simulink library "ammclib_bam_S32K14x"  (R2016a)
settings: Solver=VariableStepAuto  SolverMode=SingleTasking  StartTime=0.0  StopTime=10.0  RelTol=1e-3
undefined symbols (not defined in the file or in its folder): f16A1, f16A2, f16ADCMaxError, f16B0, f16B1, f16B2, f16C1, f16CC1, f16CC1sc, f16CC1sc_D, f16CC1sc_Q, f16CC2, f16CC2sc, f16CC2sc_D, f16CC2sc_Q, f16DerivGain, f16EGain, f16FiltCoef, f16HystOff, f16HystOn, f16IGain, f16IntegGain, f16IntegGainFW, f16IntegGainQ, f16Kd, f16Kq, f16Limit, f16LowerLimit, f16LowerLimit_D, f16LowerLimit_Q, f16LowerLimitFW, f16LowerLimitQ, f16ModIndex, f16OutValOff, f16OutValOn, f16PropGain, f16PropGainFW, f16PropGainQ, f16RampDown, f16RampUp, f16UGain, f16UpperLimit, f16UpperLimit_D, f16UpperLimit_Q, f16UpperLimitFW, f16UpperLimitQ, f16WIGain, f32A1, f32A2, f32ADCMaxError, f32B0, f32B1, f32B2, f32C1, f32CC1, f32CC1sc, f32CC1sc_D, f32CC1sc_Q, f32CC2, f32CC2sc ... (+114)
(part 22 of 22)

== system ammclib_bam_S32K14x/MLIB/FLT/MLIB_Sub_FLT ==
  fltIn1 : Inport  OutDataTypeStr=single
  fltIn2 : Inport  Port=2  OutDataTypeStr=single
  MLIB_Sub_SF : S-Function  FunctionName=MLIB_Sub_SF_FLT  SFunctionDeploymentMode=off  EnableBusSupport=off
  copyright : Subsystem
      mask Display: text(10,90,'FILE:');text(10,75,'DESRIPTION:');text(10,60,'COPYRIGHT:');text(10,45,'VERSION:');text(10,30,'DATE:')
  copyright2 : Subsystem
      mask Display: text(10,90,'MLIB_Sub_BAM_FLT.mdl');text(10,75,'Subtraction.');text(10,60,'NXP 2020');text(10,45,'1.0');text(10,30,'18-Mar-2020');
  fltOut : Outport
  wires:
  MLIB_Sub_SF/1 -> fltOut/1
  fltIn2/1 -> MLIB_Sub_SF/2
  fltIn1/1 -> MLIB_Sub_SF/1

== system ammclib_bam_S32K14x/MLIB/FLT/MLIB_VAdd_FLT ==
  fltIn1 : Inport  OutDataTypeStr=Bus: SWLIBS_2Syst_FLT  BusOutputAsStruct=on
  fltIn2 : Inport  Port=2  OutDataTypeStr=Bus: SWLIBS_2Syst_FLT  BusOutputAsStruct=on
  MLIB_VAdd_SF : S-Function  FunctionName=MLIB_VAdd_SF_FLT  SFunctionDeploymentMode=off  EnableBusSupport=off
  copyright : Subsystem
      mask Display: text(10,90,'FILE:');text(10,75,'DESRIPTION:');text(10,60,'COPYRIGHT:');text(10,45,'VERSION:');text(10,30,'DATE:')
  copyright2 : Subsystem
      mask Display: text(10,90,'MLIB_VAdd_BAM_FLT.mdl');text(10,75,'Vector addition.');text(10,60,'NXP 2020');text(10,45,'1.0');text(10,30,'28-May-2020');
  fltOut : Outport
  wires:
  MLIB_VAdd_SF/1 -> fltOut/1
  fltIn2/1 -> MLIB_VAdd_SF/2
  fltIn1/1 -> MLIB_VAdd_SF/1

== system ammclib_bam_S32K14x/MLIB/FLT/MLIB_VMac_FLT ==
  fltIn1 : Inport  OutDataTypeStr=single
  fltIn2 : Inport  Port=2  OutDataTypeStr=single
  fltIn3 : Inport  Port=3  OutDataTypeStr=single
  fltIn4 : Inport  Port=4  OutDataTypeStr=single
  MLIB_VMac_SF : S-Function  FunctionName=MLIB_VMac_SF_FLT  SFunctionDeploymentMode=off  EnableBusSupport=off
  copyright : Subsystem
      mask Display: text(10,90,'FILE:');text(10,75,'DESRIPTION:');text(10,60,'COPYRIGHT:');text(10,45,'VERSION:');text(10,30,'DATE:')
  copyright2 : Subsystem
      mask Display: text(10,90,'MLIB_VMac_BAM_FLT.mdl');text(10,75,'Dot product of 2-element vectors.');text(10,60,'NXP 2020');text(10,45,'1.0');text(10,30,'18-Mar-2020');
  fltOut : Outport
  wires:
  MLIB_VMac_SF/1 -> fltOut/1
  fltIn4/1 -> MLIB_VMac_SF/4
  fltIn3/1 -> MLIB_VMac_SF/3
  fltIn2/1 -> MLIB_VMac_SF/2
  fltIn1/1 -> MLIB_VMac_SF/1

== system ammclib_bam_S32K14x/MLIB/FLT/MLIB_VScale_FLT ==
  fltInVec : Inport  OutDataTypeStr=Bus: SWLIBS_2Syst_FLT  BusOutputAsStruct=on
  fltInScale : Inport  Port=2  OutDataTypeStr=single
  MLIB_VScale_SF : S-Function  FunctionName=MLIB_VScale_SF_FLT  SFunctionDeploymentMode=off  EnableBusSupport=off
  copyright : Subsystem
      mask Display: text(10,90,'FILE:');text(10,75,'DESRIPTION:');text(10,60,'COPYRIGHT:');text(10,45,'VERSION:');text(10,30,'DATE:')
  copyright2 : Subsystem
      mask Display: text(10,90,'MLIB_VScale_BAM_FLT.mdl');text(10,75,'Multiplication of a vector and scalar.');text(10,60,'NXP 2020');text(10,45,'1.0');text(10,30,'03-Jun-2020');
  fltOutVec : Outport
  wires:
  MLIB_VScale_SF/1 -> fltOutVec/1
  fltInScale/1 -> MLIB_VScale_SF/2
  fltInVec/1 -> MLIB_VScale_SF/1

== system ammclib_bam_S32K14x/MLIB/FLT/MLIB_VSub_FLT ==
  fltIn1 : Inport  OutDataTypeStr=Bus: SWLIBS_2Syst_FLT  BusOutputAsStruct=on
  fltIn2 : Inport  Port=2  OutDataTypeStr=Bus: SWLIBS_2Syst_FLT  BusOutputAsStruct=on
  MLIB_VSub_SF : S-Function  FunctionName=MLIB_VSub_SF_FLT  SFunctionDeploymentMode=off  EnableBusSupport=off
  copyright : Subsystem
      mask Display: text(10,90,'FILE:');text(10,75,'DESRIPTION:');text(10,60,'COPYRIGHT:');text(10,45,'VERSION:');text(10,30,'DATE:')
  copyright2 : Subsystem
      mask Display: text(10,90,'MLIB_VSub_BAM_FLT.mdl');text(10,75,'Vector substraction.');text(10,60,'NXP 2020');text(10,45,'1.0');text(10,30,'01-Jun-2020');
  fltOut : Outport
  wires:
  MLIB_VSub_SF/1 -> fltOut/1
  fltIn2/1 -> MLIB_VSub_SF/2
  fltIn1/1 -> MLIB_VSub_SF/1

== system ammclib_bam_S32K14x/AMCLIB/F16/AMCLIB_BemfObsrvDQ_F16/copyright ==

== system ammclib_bam_S32K14x/AMCLIB/F16/AMCLIB_BemfObsrvDQ_F16/copyright2 ==

== system ammclib_bam_S32K14x/AMCLIB/F16/AMCLIB_CurrentLoop_F16/copyright ==

== system ammclib_bam_S32K14x/AMCLIB/F16/AMCLIB_CurrentLoop_F16/copyright2 ==

== system ammclib_bam_S32K14x/AMCLIB/F16/AMCLIB_FWSpeedLoop_F16/copyright ==

== system ammclib_bam_S32K14x/AMCLIB/F16/AMCLIB_FWSpeedLoop_F16/copyright2 ==

== system ammclib_bam_S32K14x/AMCLIB/F16/AMCLIB_FW_F16/copyright ==

== system ammclib_bam_S32K14x/AMCLIB/F16/AMCLIB_FW_F16/copyright2 ==

== system ammclib_bam_S32K14x/AMCLIB/F16/AMCLIB_SpeedLoop_F16/copyright ==

== system ammclib_bam_S32K14x/AMCLIB/F16/AMCLIB_SpeedLoop_F16/copyright2 ==

== system ammclib_bam_S32K14x/AMCLIB/F16/AMCLIB_TrackObsrv_F16/copyright ==

== system ammclib_bam_S32K14x/AMCLIB/F16/AMCLIB_TrackObsrv_F16/copyright2 ==

== system ammclib_bam_S32K14x/AMCLIB/F16/AMCLIB_Windmilling_F16/copyright ==

== system ammclib_bam_S32K14x/AMCLIB/F16/AMCLIB_Windmilling_F16/copyright2 ==

== system ammclib_bam_S32K14x/AMCLIB/F32/AMCLIB_BemfObsrvDQ_F32/copyright ==

== system ammclib_bam_S32K14x/AMCLIB/F32/AMCLIB_BemfObsrvDQ_F32/copyright2 ==

== system ammclib_bam_S32K14x/AMCLIB/F32/AMCLIB_CurrentLoop_F32/copyright ==

== system ammclib_bam_S32K14x/AMCLIB/F32/AMCLIB_CurrentLoop_F32/copyright2 ==

== system ammclib_bam_S32K14x/AMCLIB/F32/AMCLIB_FWSpeedLoop_F32/copyright ==

== system ammclib_bam_S32K14x/AMCLIB/F32/AMCLIB_FWSpeedLoop_F32/copyright2 ==

== system ammclib_bam_S32K14x/AMCLIB/F32/AMCLIB_FW_F32/copyright ==

== system ammclib_bam_S32K14x/AMCLIB/F32/AMCLIB_FW_F32/copyright2 ==

== system ammclib_bam_S32K14x/AMCLIB/F32/AMCLIB_SpeedLoop_F32/copyright ==

== system ammclib_bam_S32K14x/AMCLIB/F32/AMCLIB_SpeedLoop_F32/copyright2 ==

== system ammclib_bam_S32K14x/AMCLIB/F32/AMCLIB_TrackObsrv_F32/copyright ==

== system ammclib_bam_S32K14x/AMCLIB/F32/AMCLIB_TrackObsrv_F32/copyright2 ==

== system ammclib_bam_S32K14x/AMCLIB/F32/AMCLIB_Windmilling_F32/copyright ==

== system ammclib_bam_S32K14x/AMCLIB/F32/AMCLIB_Windmilling_F32/copyright2 ==

== system ammclib_bam_S32K14x/AMCLIB/FLT/AMCLIB_BemfObsrvDQ_FLT/copyright ==

== system ammclib_bam_S32K14x/AMCLIB/FLT/AMCLIB_BemfObsrvDQ_FLT/copyright2 ==

== system ammclib_bam_S32K14x/AMCLIB/FLT/AMCLIB_CurrentLoop_FLT/copyright ==

== system ammclib_bam_S32K14x/AMCLIB/FLT/AMCLIB_CurrentLoop_FLT/copyright2 ==

== system ammclib_bam_S32K14x/AMCLIB/FLT/AMCLIB_FWSpeedLoop_FLT/copyright ==

== system ammclib_bam_S32K14x/AMCLIB/FLT/AMCLIB_FWSpeedLoop_FLT/copyright2 ==

== system ammclib_bam_S32K14x/AMCLIB/FLT/AMCLIB_FW_FLT/copyright ==

== system ammclib_bam_S32K14x/AMCLIB/FLT/AMCLIB_FW_FLT/copyright2 ==

== system ammclib_bam_S32K14x/AMCLIB/FLT/AMCLIB_SpeedLoop_FLT/copyright ==

== system ammclib_bam_S32K14x/AMCLIB/FLT/AMCLIB_SpeedLoop_FLT/copyright2 ==

== system ammclib_bam_S32K14x/AMCLIB/FLT/AMCLIB_TrackObsrv_FLT/copyright ==

== system ammclib_bam_S32K14x/AMCLIB/FLT/AMCLIB_TrackObsrv_FLT/copyright2 ==

== system ammclib_bam_S32K14x/AMCLIB/FLT/AMCLIB_Windmilling_FLT/copyright ==

== system ammclib_bam_S32K14x/AMCLIB/FLT/AMCLIB_Windmilling_FLT/copyright2 ==

== system ammclib_bam_S32K14x/GDFLIB/F16/GDFLIB_FilterFIR_F16/copyright ==

== system ammclib_bam_S32K14x/GDFLIB/F16/GDFLIB_FilterFIR_F16/copyright2 ==

== system ammclib_bam_S32K14x/GDFLIB/F16/GDFLIB_FilterIIR1_F16/copyright ==

== system ammclib_bam_S32K14x/GDFLIB/F16/GDFLIB_FilterIIR1_F16/copyright2 ==

== system ammclib_bam_S32K14x/GDFLIB/F16/GDFLIB_FilterIIR2_F16/copyright ==

== system ammclib_bam_S32K14x/GDFLIB/F16/GDFLIB_FilterIIR2_F16/copyright2 ==

== system ammclib_bam_S32K14x/GDFLIB/F16/GDFLIB_FilterMA_F16/copyright ==

== system ammclib_bam_S32K14x/GDFLIB/F16/GDFLIB_FilterMA_F16/copyright2 ==

== system ammclib_bam_S32K14x/GDFLIB/F32/GDFLIB_FilterFIR_F32/copyright ==

== system ammclib_bam_S32K14x/GDFLIB/F32/GDFLIB_FilterFIR_F32/copyright2 ==

== system ammclib_bam_S32K14x/GDFLIB/F32/GDFLIB_FilterIIR1_F32/copyright ==

== system ammclib_bam_S32K14x/GDFLIB/F32/GDFLIB_FilterIIR1_F32/copyright2 ==

== system ammclib_bam_S32K14x/GDFLIB/F32/GDFLIB_FilterIIR2_F32/copyright ==

== system ammclib_bam_S32K14x/GDFLIB/F32/GDFLIB_FilterIIR2_F32/copyright2 ==

== system ammclib_bam_S32K14x/GDFLIB/F32/GDFLIB_FilterMA_F32/copyright ==

== system ammclib_bam_S32K14x/GDFLIB/F32/GDFLIB_FilterMA_F32/copyright2 ==

== system ammclib_bam_S32K14x/GDFLIB/FLT/GDFLIB_FilterFIR_FLT/copyright ==

== system ammclib_bam_S32K14x/GDFLIB/FLT/GDFLIB_FilterFIR_FLT/copyright2 ==

== system ammclib_bam_S32K14x/GDFLIB/FLT/GDFLIB_FilterIIR1_FLT/copyright ==

== system ammclib_bam_S32K14x/GDFLIB/FLT/GDFLIB_FilterIIR1_FLT/copyright2 ==

== system ammclib_bam_S32K14x/GDFLIB/FLT/GDFLIB_FilterIIR2_FLT/copyright ==

== system ammclib_bam_S32K14x/GDFLIB/FLT/GDFLIB_FilterIIR2_FLT/copyright2 ==

== system ammclib_bam_S32K14x/GDFLIB/FLT/GDFLIB_FilterMA_FLT/copyright ==

== system ammclib_bam_S32K14x/GDFLIB/FLT/GDFLIB_FilterMA_FLT/copyright2 ==

== system ammclib_bam_S32K14x/GFLIB/F16/GFLIB_Acos_F16/copyright ==

== system ammclib_bam_S32K14x/GFLIB/F16/GFLIB_Acos_F16/copyright2 ==

== system ammclib_bam_S32K14x/GFLIB/F16/GFLIB_Asin_F16/copyright ==

== system ammclib_bam_S32K14x/GFLIB/F16/GFLIB_Asin_F16/copyright2 ==

== system ammclib_bam_S32K14x/GFLIB/F16/GFLIB_AtanYXShifted_F16/copyright ==

== system ammclib_bam_S32K14x/GFLIB/F16/GFLIB_AtanYXShifted_F16/copyright2 ==

== system ammclib_bam_S32K14x/GFLIB/F16/GFLIB_AtanYX_F16/copyright ==

== system ammclib_bam_S32K14x/GFLIB/F16/GFLIB_AtanYX_F16/copyright2 ==

== system ammclib_bam_S32K14x/GFLIB/F16/GFLIB_Atan_F16/copyright ==

== system ammclib_bam_S32K14x/GFLIB/F16/GFLIB_Atan_F16/copyright2 ==

== system ammclib_bam_S32K14x/GFLIB/F16/GFLIB_ControllerPIDpAW_F16/copyright ==

== system ammclib_bam_S32K14x/GFLIB/F16/GFLIB_ControllerPIDpAW_F16/copyright2 ==

== system ammclib_bam_S32K14x/GFLIB/F16/GFLIB_ControllerPIpAW_F16/copyright ==

== system ammclib_bam_S32K14x/GFLIB/F16/GFLIB_ControllerPIpAW_F16/copyright2 ==

== system ammclib_bam_S32K14x/GFLIB/F16/GFLIB_ControllerPIp_F16/copyright ==

== system ammclib_bam_S32K14x/GFLIB/F16/GFLIB_ControllerPIp_F16/copyright2 ==

== system ammclib_bam_S32K14x/GFLIB/F16/GFLIB_ControllerPIrAW_F16/copyright ==

== system ammclib_bam_S32K14x/GFLIB/F16/GFLIB_ControllerPIrAW_F16/copyright2 ==

== system ammclib_bam_S32K14x/GFLIB/F16/GFLIB_ControllerPIr_F16/copyright ==

== system ammclib_bam_S32K14x/GFLIB/F16/GFLIB_ControllerPIr_F16/copyright2 ==

== system ammclib_bam_S32K14x/GFLIB/F16/GFLIB_Cos_F16/copyright ==

== system ammclib_bam_S32K14x/GFLIB/F16/GFLIB_Cos_F16/copyright2 ==

== system ammclib_bam_S32K14x/GFLIB/F16/GFLIB_Hyst_F16/copyright ==

== system ammclib_bam_S32K14x/GFLIB/F16/GFLIB_Hyst_F16/copyright2 ==

== system ammclib_bam_S32K14x/GFLIB/F16/GFLIB_IntegratorTR_F16/copyright ==

== system ammclib_bam_S32K14x/GFLIB/F16/GFLIB_IntegratorTR_F16/copyright2 ==

== system ammclib_bam_S32K14x/GFLIB/F16/GFLIB_Limit_F16/copyright ==

== system ammclib_bam_S32K14x/GFLIB/F16/GFLIB_Limit_F16/copyright2 ==

== system ammclib_bam_S32K14x/GFLIB/F16/GFLIB_LowerLimit_F16/copyright ==

== system ammclib_bam_S32K14x/GFLIB/F16/GFLIB_LowerLimit_F16/copyright2 ==

== system ammclib_bam_S32K14x/GFLIB/F16/GFLIB_Lut1D_F16/copyright ==

== system ammclib_bam_S32K14x/GFLIB/F16/GFLIB_Lut1D_F16/copyright2 ==

== system ammclib_bam_S32K14x/GFLIB/F16/GFLIB_Lut2D_F16/copyright ==

== system ammclib_bam_S32K14x/GFLIB/F16/GFLIB_Lut2D_F16/copyright2 ==

== system ammclib_bam_S32K14x/GFLIB/F16/GFLIB_Ramp_F16/copyright ==

== system ammclib_bam_S32K14x/GFLIB/F16/GFLIB_Ramp_F16/copyright2 ==

== system ammclib_bam_S32K14x/GFLIB/F16/GFLIB_Sign_F16/copyright ==

== system ammclib_bam_S32K14x/GFLIB/F16/GFLIB_Sign_F16/copyright2 ==

== system ammclib_bam_S32K14x/GFLIB/F16/GFLIB_SinCos_F16/copyright ==

== system ammclib_bam_S32K14x/GFLIB/F16/GFLIB_SinCos_F16/copyright2 ==

== system ammclib_bam_S32K14x/GFLIB/F16/GFLIB_Sin_F16/copyright ==

== system ammclib_bam_S32K14x/GFLIB/F16/GFLIB_Sin_F16/copyright2 ==

== system ammclib_bam_S32K14x/GFLIB/F16/GFLIB_Sqrt_F16/copyright ==

== system ammclib_bam_S32K14x/GFLIB/F16/GFLIB_Sqrt_F16/copyright2 ==

== system ammclib_bam_S32K14x/GFLIB/F16/GFLIB_Tan_F16/copyright ==

== system ammclib_bam_S32K14x/GFLIB/F16/GFLIB_Tan_F16/copyright2 ==

== system ammclib_bam_S32K14x/GFLIB/F16/GFLIB_UpperLimit_F16/copyright ==

== system ammclib_bam_S32K14x/GFLIB/F16/GFLIB_UpperLimit_F16/copyright2 ==

== system ammclib_bam_S32K14x/GFLIB/F16/GFLIB_VMin_F16/copyright ==

== system ammclib_bam_S32K14x/GFLIB/F16/GFLIB_VMin_F16/copyright2 ==

== system ammclib_bam_S32K14x/GFLIB/F16/GFLIB_VectorLimit_F16/copyright ==

== system ammclib_bam_S32K14x/GFLIB/F16/GFLIB_VectorLimit_F16/copyright2 ==

== system ammclib_bam_S32K14x/GFLIB/F32/GFLIB_Acos_F32/copyright ==

== system ammclib_bam_S32K14x/GFLIB/F32/GFLIB_Acos_F32/copyright2 ==

== system ammclib_bam_S32K14x/GFLIB/F32/GFLIB_Asin_F32/copyright ==

== system ammclib_bam_S32K14x/GFLIB/F32/GFLIB_Asin_F32/copyright2 ==

== system ammclib_bam_S32K14x/GFLIB/F32/GFLIB_AtanYXShifted_F32/copyright ==

== system ammclib_bam_S32K14x/GFLIB/F32/GFLIB_AtanYXShifted_F32/copyright2 ==

== system ammclib_bam_S32K14x/GFLIB/F32/GFLIB_AtanYX_F32/copyright ==

== system ammclib_bam_S32K14x/GFLIB/F32/GFLIB_AtanYX_F32/copyright2 ==

== system ammclib_bam_S32K14x/GFLIB/F32/GFLIB_Atan_F32/copyright ==

== system ammclib_bam_S32K14x/GFLIB/F32/GFLIB_Atan_F32/copyright2 ==

== system ammclib_bam_S32K14x/GFLIB/F32/GFLIB_ControllerPIDpAW_F32/copyright ==

== system ammclib_bam_S32K14x/GFLIB/F32/GFLIB_ControllerPIDpAW_F32/copyright2 ==

== system ammclib_bam_S32K14x/GFLIB/F32/GFLIB_ControllerPIpAW_F32/copyright ==

== system ammclib_bam_S32K14x/GFLIB/F32/GFLIB_ControllerPIpAW_F32/copyright2 ==

== system ammclib_bam_S32K14x/GFLIB/F32/GFLIB_ControllerPIp_F32/copyright ==

== system ammclib_bam_S32K14x/GFLIB/F32/GFLIB_ControllerPIp_F32/copyright2 ==

== system ammclib_bam_S32K14x/GFLIB/F32/GFLIB_ControllerPIrAW_F32/copyright ==

== system ammclib_bam_S32K14x/GFLIB/F32/GFLIB_ControllerPIrAW_F32/copyright2 ==

== system ammclib_bam_S32K14x/GFLIB/F32/GFLIB_ControllerPIr_F32/copyright ==

== system ammclib_bam_S32K14x/GFLIB/F32/GFLIB_ControllerPIr_F32/copyright2 ==

== system ammclib_bam_S32K14x/GFLIB/F32/GFLIB_Cos_F32/copyright ==

== system ammclib_bam_S32K14x/GFLIB/F32/GFLIB_Cos_F32/copyright2 ==

== system ammclib_bam_S32K14x/GFLIB/F32/GFLIB_Hyst_F32/copyright ==

== system ammclib_bam_S32K14x/GFLIB/F32/GFLIB_Hyst_F32/copyright2 ==

== system ammclib_bam_S32K14x/GFLIB/F32/GFLIB_IntegratorTR_F32/copyright ==

== system ammclib_bam_S32K14x/GFLIB/F32/GFLIB_IntegratorTR_F32/copyright2 ==

== system ammclib_bam_S32K14x/GFLIB/F32/GFLIB_Limit_F32/copyright ==

== system ammclib_bam_S32K14x/GFLIB/F32/GFLIB_Limit_F32/copyright2 ==

== system ammclib_bam_S32K14x/GFLIB/F32/GFLIB_LowerLimit_F32/copyright ==

== system ammclib_bam_S32K14x/GFLIB/F32/GFLIB_LowerLimit_F32/copyright2 ==

== system ammclib_bam_S32K14x/GFLIB/F32/GFLIB_Lut1D_F32/copyright ==

== system ammclib_bam_S32K14x/GFLIB/F32/GFLIB_Lut1D_F32/copyright2 ==

== system ammclib_bam_S32K14x/GFLIB/F32/GFLIB_Lut2D_F32/copyright ==

== system ammclib_bam_S32K14x/GFLIB/F32/GFLIB_Lut2D_F32/copyright2 ==

== system ammclib_bam_S32K14x/GFLIB/F32/GFLIB_Ramp_F32/copyright ==

== system ammclib_bam_S32K14x/GFLIB/F32/GFLIB_Ramp_F32/copyright2 ==

== system ammclib_bam_S32K14x/GFLIB/F32/GFLIB_Sign_F32/copyright ==

== system ammclib_bam_S32K14x/GFLIB/F32/GFLIB_Sign_F32/copyright2 ==

== system ammclib_bam_S32K14x/GFLIB/F32/GFLIB_SinCos_F32/copyright ==

== system ammclib_bam_S32K14x/GFLIB/F32/GFLIB_SinCos_F32/copyright2 ==

== system ammclib_bam_S32K14x/GFLIB/F32/GFLIB_Sin_F32/copyright ==

== system ammclib_bam_S32K14x/GFLIB/F32/GFLIB_Sin_F32/copyright2 ==

== system ammclib_bam_S32K14x/GFLIB/F32/GFLIB_Sqrt_F32/copyright ==

== system ammclib_bam_S32K14x/GFLIB/F32/GFLIB_Sqrt_F32/copyright2 ==

== system ammclib_bam_S32K14x/GFLIB/F32/GFLIB_Tan_F32/copyright ==

== system ammclib_bam_S32K14x/GFLIB/F32/GFLIB_Tan_F32/copyright2 ==

== system ammclib_bam_S32K14x/GFLIB/F32/GFLIB_UpperLimit_F32/copyright ==

== system ammclib_bam_S32K14x/GFLIB/F32/GFLIB_UpperLimit_F32/copyright2 ==

== system ammclib_bam_S32K14x/GFLIB/F32/GFLIB_VMin_F32/copyright ==

== system ammclib_bam_S32K14x/GFLIB/F32/GFLIB_VMin_F32/copyright2 ==

== system ammclib_bam_S32K14x/GFLIB/F32/GFLIB_VectorLimit_F32/copyright ==

== system ammclib_bam_S32K14x/GFLIB/F32/GFLIB_VectorLimit_F32/copyright2 ==

== system ammclib_bam_S32K14x/GFLIB/FLT/GFLIB_Acos_FLT/copyright ==

== system ammclib_bam_S32K14x/GFLIB/FLT/GFLIB_Acos_FLT/copyright2 ==

== system ammclib_bam_S32K14x/GFLIB/FLT/GFLIB_Asin_FLT/copyright ==

== system ammclib_bam_S32K14x/GFLIB/FLT/GFLIB_Asin_FLT/copyright2 ==

== system ammclib_bam_S32K14x/GFLIB/FLT/GFLIB_AtanYXShifted_FLT/copyright ==

== system ammclib_bam_S32K14x/GFLIB/FLT/GFLIB_AtanYXShifted_FLT/copyright2 ==

== system ammclib_bam_S32K14x/GFLIB/FLT/GFLIB_AtanYX_FLT/copyright ==

== system ammclib_bam_S32K14x/GFLIB/FLT/GFLIB_AtanYX_FLT/copyright2 ==

== system ammclib_bam_S32K14x/GFLIB/FLT/GFLIB_Atan_FLT/copyright ==

== system ammclib_bam_S32K14x/GFLIB/FLT/GFLIB_Atan_FLT/copyright2 ==

== system ammclib_bam_S32K14x/GFLIB/FLT/GFLIB_ControllerPIDpAW_FLT/copyright ==

== system ammclib_bam_S32K14x/GFLIB/FLT/GFLIB_ControllerPIDpAW_FLT/copyright2 ==

== system ammclib_bam_S32K14x/GFLIB/FLT/GFLIB_ControllerPIpAW_FLT/copyright ==

== system ammclib_bam_S32K14x/GFLIB/FLT/GFLIB_ControllerPIpAW_FLT/copyright2 ==

== system ammclib_bam_S32K14x/GFLIB/FLT/GFLIB_ControllerPIp_FLT/copyright ==

== system ammclib_bam_S32K14x/GFLIB/FLT/GFLIB_ControllerPIp_FLT/copyright2 ==

== system ammclib_bam_S32K14x/GFLIB/FLT/GFLIB_ControllerPIrAW_FLT/copyright ==

== system ammclib_bam_S32K14x/GFLIB/FLT/GFLIB_ControllerPIrAW_FLT/copyright2 ==

== system ammclib_bam_S32K14x/GFLIB/FLT/GFLIB_ControllerPIr_FLT/copyright ==

== system ammclib_bam_S32K14x/GFLIB/FLT/GFLIB_ControllerPIr_FLT/copyright2 ==

== system ammclib_bam_S32K14x/GFLIB/FLT/GFLIB_Cos_FLT/copyright ==

== system ammclib_bam_S32K14x/GFLIB/FLT/GFLIB_Cos_FLT/copyright2 ==

== system ammclib_bam_S32K14x/GFLIB/FLT/GFLIB_Hyst_FLT/copyright ==

== system ammclib_bam_S32K14x/GFLIB/FLT/GFLIB_Hyst_FLT/copyright2 ==

== system ammclib_bam_S32K14x/GFLIB/FLT/GFLIB_IntegratorTR_FLT/copyright ==

== system ammclib_bam_S32K14x/GFLIB/FLT/GFLIB_IntegratorTR_FLT/copyright2 ==

== system ammclib_bam_S32K14x/GFLIB/FLT/GFLIB_Limit_FLT/copyright ==

== system ammclib_bam_S32K14x/GFLIB/FLT/GFLIB_Limit_FLT/copyright2 ==

== system ammclib_bam_S32K14x/GFLIB/FLT/GFLIB_Log10_FLT/copyright ==

== system ammclib_bam_S32K14x/GFLIB/FLT/GFLIB_Log10_FLT/copyright2 ==

== system ammclib_bam_S32K14x/GFLIB/FLT/GFLIB_LowerLimit_FLT/copyright ==

== system ammclib_bam_S32K14x/GFLIB/FLT/GFLIB_LowerLimit_FLT/copyright2 ==

== system ammclib_bam_S32K14x/GFLIB/FLT/GFLIB_Lut1D_FLT/copyright ==

== system ammclib_bam_S32K14x/GFLIB/FLT/GFLIB_Lut1D_FLT/copyright2 ==

== system ammclib_bam_S32K14x/GFLIB/FLT/GFLIB_Lut2D_FLT/copyright ==

== system ammclib_bam_S32K14x/GFLIB/FLT/GFLIB_Lut2D_FLT/copyright2 ==

== system ammclib_bam_S32K14x/GFLIB/FLT/GFLIB_Ramp_FLT/copyright ==

== system ammclib_bam_S32K14x/GFLIB/FLT/GFLIB_Ramp_FLT/copyright2 ==

== system ammclib_bam_S32K14x/GFLIB/FLT/GFLIB_Sign_FLT/copyright ==

== system ammclib_bam_S32K14x/GFLIB/FLT/GFLIB_Sign_FLT/copyright2 ==

== system ammclib_bam_S32K14x/GFLIB/FLT/GFLIB_SinCos_FLT/copyright ==

== system ammclib_bam_S32K14x/GFLIB/FLT/GFLIB_SinCos_FLT/copyright2 ==

== system ammclib_bam_S32K14x/GFLIB/FLT/GFLIB_Sin_FLT/copyright ==

== system ammclib_bam_S32K14x/GFLIB/FLT/GFLIB_Sin_FLT/copyright2 ==

== system ammclib_bam_S32K14x/GFLIB/FLT/GFLIB_Sqrt_FLT/copyright ==

== system ammclib_bam_S32K14x/GFLIB/FLT/GFLIB_Sqrt_FLT/copyright2 ==

== system ammclib_bam_S32K14x/GFLIB/FLT/GFLIB_Tan_FLT/copyright ==

== system ammclib_bam_S32K14x/GFLIB/FLT/GFLIB_Tan_FLT/copyright2 ==

== system ammclib_bam_S32K14x/GFLIB/FLT/GFLIB_UpperLimit_FLT/copyright ==

== system ammclib_bam_S32K14x/GFLIB/FLT/GFLIB_UpperLimit_FLT/copyright2 ==

== system ammclib_bam_S32K14x/GFLIB/FLT/GFLIB_VLog10_FLT/copyright ==

== system ammclib_bam_S32K14x/GFLIB/FLT/GFLIB_VLog10_FLT/copyright2 ==

== system ammclib_bam_S32K14x/GFLIB/FLT/GFLIB_VMin_FLT/copyright ==

== system ammclib_bam_S32K14x/GFLIB/FLT/GFLIB_VMin_FLT/copyright2 ==

== system ammclib_bam_S32K14x/GFLIB/FLT/GFLIB_VectorLimit_FLT/copyright ==

== system ammclib_bam_S32K14x/GFLIB/FLT/GFLIB_VectorLimit_FLT/copyright2 ==

== system ammclib_bam_S32K14x/GMCLIB/F16/GMCLIB_BetaProjection3Ph_F16/copyright ==

== system ammclib_bam_S32K14x/GMCLIB/F16/GMCLIB_BetaProjection3Ph_F16/copyright2 ==

== system ammclib_bam_S32K14x/GMCLIB/F16/GMCLIB_BetaProjection_F16/copyright ==

== system ammclib_bam_S32K14x/GMCLIB/F16/GMCLIB_BetaProjection_F16/copyright2 ==

== system ammclib_bam_S32K14x/GMCLIB/F16/GMCLIB_ClarkInv_F16/copyright ==

== system ammclib_bam_S32K14x/GMCLIB/F16/GMCLIB_ClarkInv_F16/copyright2 ==

== system ammclib_bam_S32K14x/GMCLIB/F16/GMCLIB_Clark_F16/copyright ==

== system ammclib_bam_S32K14x/GMCLIB/F16/GMCLIB_Clark_F16/copyright2 ==

== system ammclib_bam_S32K14x/GMCLIB/F16/GMCLIB_DecouplingPMSM_F16/copyright ==

== system ammclib_bam_S32K14x/GMCLIB/F16/GMCLIB_DecouplingPMSM_F16/copyright2 ==

== system ammclib_bam_S32K14x/GMCLIB/F16/GMCLIB_ElimDcBusRip_F16/copyright ==

== system ammclib_bam_S32K14x/GMCLIB/F16/GMCLIB_ElimDcBusRip_F16/copyright2 ==

== system ammclib_bam_S32K14x/GMCLIB/F16/GMCLIB_ParkInv_F16/copyright ==

== system ammclib_bam_S32K14x/GMCLIB/F16/GMCLIB_ParkInv_F16/copyright2 ==

== system ammclib_bam_S32K14x/GMCLIB/F16/GMCLIB_Park_F16/copyright ==

== system ammclib_bam_S32K14x/GMCLIB/F16/GMCLIB_Park_F16/copyright2 ==

== system ammclib_bam_S32K14x/GMCLIB/F16/GMCLIB_PwmIct_F16/copyright ==

== system ammclib_bam_S32K14x/GMCLIB/F16/GMCLIB_PwmIct_F16/copyright2 ==

== system ammclib_bam_S32K14x/GMCLIB/F16/GMCLIB_SvmSci_F16/copyright ==

== system ammclib_bam_S32K14x/GMCLIB/F16/GMCLIB_SvmSci_F16/copyright2 ==

== system ammclib_bam_S32K14x/GMCLIB/F16/GMCLIB_SvmStd_F16/copyright ==

== system ammclib_bam_S32K14x/GMCLIB/F16/GMCLIB_SvmStd_F16/copyright2 ==

== system ammclib_bam_S32K14x/GMCLIB/F16/GMCLIB_SvmU0n_F16/copyright ==

== system ammclib_bam_S32K14x/GMCLIB/F16/GMCLIB_SvmU0n_F16/copyright2 ==

== system ammclib_bam_S32K14x/GMCLIB/F16/GMCLIB_SvmU7n_F16/copyright ==

== system ammclib_bam_S32K14x/GMCLIB/F16/GMCLIB_SvmU7n_F16/copyright2 ==

== system ammclib_bam_S32K14x/GMCLIB/F16/GMCLIB_VRot_F16/copyright ==

== system ammclib_bam_S32K14x/GMCLIB/F16/GMCLIB_VRot_F16/copyright2 ==

== system ammclib_bam_S32K14x/GMCLIB/F16/GMCLIB_VUnit_F16/copyright ==

== system ammclib_bam_S32K14x/GMCLIB/F16/GMCLIB_VUnit_F16/copyright2 ==

== system ammclib_bam_S32K14x/GMCLIB/F16/GMCLIB_Vpol2xy_F16/copyright ==

== system ammclib_bam_S32K14x/GMCLIB/F16/GMCLIB_Vpol2xy_F16/copyright2 ==

== system ammclib_bam_S32K14x/GMCLIB/F16/GMCLIB_Vxy2pol_F16/copyright ==

== system ammclib_bam_S32K14x/GMCLIB/F16/GMCLIB_Vxy2pol_F16/copyright2 ==

== system ammclib_bam_S32K14x/GMCLIB/F32/GMCLIB_BetaProjection3Ph_F32/copyright ==

== system ammclib_bam_S32K14x/GMCLIB/F32/GMCLIB_BetaProjection3Ph_F32/copyright2 ==

== system ammclib_bam_S32K14x/GMCLIB/F32/GMCLIB_BetaProjection_F32/copyright ==

== system ammclib_bam_S32K14x/GMCLIB/F32/GMCLIB_BetaProjection_F32/copyright2 ==

== system ammclib_bam_S32K14x/GMCLIB/F32/GMCLIB_ClarkInv_F32/copyright ==

== system ammclib_bam_S32K14x/GMCLIB/F32/GMCLIB_ClarkInv_F32/copyright2 ==

== system ammclib_bam_S32K14x/GMCLIB/F32/GMCLIB_Clark_F32/copyright ==

== system ammclib_bam_S32K14x/GMCLIB/F32/GMCLIB_Clark_F32/copyright2 ==

== system ammclib_bam_S32K14x/GMCLIB/F32/GMCLIB_DecouplingPMSM_F32/copyright ==

== system ammclib_bam_S32K14x/GMCLIB/F32/GMCLIB_DecouplingPMSM_F32/copyright2 ==

== system ammclib_bam_S32K14x/GMCLIB/F32/GMCLIB_ElimDcBusRip_F32/copyright ==

== system ammclib_bam_S32K14x/GMCLIB/F32/GMCLIB_ElimDcBusRip_F32/copyright2 ==

== system ammclib_bam_S32K14x/GMCLIB/F32/GMCLIB_ParkInv_F32/copyright ==

== system ammclib_bam_S32K14x/GMCLIB/F32/GMCLIB_ParkInv_F32/copyright2 ==

== system ammclib_bam_S32K14x/GMCLIB/F32/GMCLIB_Park_F32/copyright ==

== system ammclib_bam_S32K14x/GMCLIB/F32/GMCLIB_Park_F32/copyright2 ==

== system ammclib_bam_S32K14x/GMCLIB/F32/GMCLIB_PwmIct_F32/copyright ==

== system ammclib_bam_S32K14x/GMCLIB/F32/GMCLIB_PwmIct_F32/copyright2 ==

== system ammclib_bam_S32K14x/GMCLIB/F32/GMCLIB_SvmSci_F32/copyright ==

== system ammclib_bam_S32K14x/GMCLIB/F32/GMCLIB_SvmSci_F32/copyright2 ==

== system ammclib_bam_S32K14x/GMCLIB/F32/GMCLIB_SvmStd_F32/copyright ==

== system ammclib_bam_S32K14x/GMCLIB/F32/GMCLIB_SvmStd_F32/copyright2 ==

== system ammclib_bam_S32K14x/GMCLIB/F32/GMCLIB_SvmU0n_F32/copyright ==

== system ammclib_bam_S32K14x/GMCLIB/F32/GMCLIB_SvmU0n_F32/copyright2 ==

== system ammclib_bam_S32K14x/GMCLIB/F32/GMCLIB_SvmU7n_F32/copyright ==

== system ammclib_bam_S32K14x/GMCLIB/F32/GMCLIB_SvmU7n_F32/copyright2 ==

== system ammclib_bam_S32K14x/GMCLIB/F32/GMCLIB_VRot_F32/copyright ==

== system ammclib_bam_S32K14x/GMCLIB/F32/GMCLIB_VRot_F32/copyright2 ==

== system ammclib_bam_S32K14x/GMCLIB/F32/GMCLIB_VUnit_F32/copyright ==

== system ammclib_bam_S32K14x/GMCLIB/F32/GMCLIB_VUnit_F32/copyright2 ==

== system ammclib_bam_S32K14x/GMCLIB/F32/GMCLIB_Vpol2xy_F32/copyright ==

== system ammclib_bam_S32K14x/GMCLIB/F32/GMCLIB_Vpol2xy_F32/copyright2 ==

== system ammclib_bam_S32K14x/GMCLIB/F32/GMCLIB_Vxy2pol_F32/copyright ==

== system ammclib_bam_S32K14x/GMCLIB/F32/GMCLIB_Vxy2pol_F32/copyright2 ==

== system ammclib_bam_S32K14x/GMCLIB/FLT/GMCLIB_BetaProjection3Ph_FLT/copyright ==

== system ammclib_bam_S32K14x/GMCLIB/FLT/GMCLIB_BetaProjection3Ph_FLT/copyright2 ==

== system ammclib_bam_S32K14x/GMCLIB/FLT/GMCLIB_BetaProjection_FLT/copyright ==

== system ammclib_bam_S32K14x/GMCLIB/FLT/GMCLIB_BetaProjection_FLT/copyright2 ==

== system ammclib_bam_S32K14x/GMCLIB/FLT/GMCLIB_ClarkInv_FLT/copyright ==

== system ammclib_bam_S32K14x/GMCLIB/FLT/GMCLIB_ClarkInv_FLT/copyright2 ==

== system ammclib_bam_S32K14x/GMCLIB/FLT/GMCLIB_Clark_FLT/copyright ==

== system ammclib_bam_S32K14x/GMCLIB/FLT/GMCLIB_Clark_FLT/copyright2 ==

== system ammclib_bam_S32K14x/GMCLIB/FLT/GMCLIB_DecouplingPMSM_FLT/copyright ==

== system ammclib_bam_S32K14x/GMCLIB/FLT/GMCLIB_DecouplingPMSM_FLT/copyright2 ==

== system ammclib_bam_S32K14x/GMCLIB/FLT/GMCLIB_ElimDcBusRip_FLT/copyright ==

== system ammclib_bam_S32K14x/GMCLIB/FLT/GMCLIB_ElimDcBusRip_FLT/copyright2 ==

== system ammclib_bam_S32K14x/GMCLIB/FLT/GMCLIB_ParkInv_FLT/copyright ==

== system ammclib_bam_S32K14x/GMCLIB/FLT/GMCLIB_ParkInv_FLT/copyright2 ==

== system ammclib_bam_S32K14x/GMCLIB/FLT/GMCLIB_Park_FLT/copyright ==

== system ammclib_bam_S32K14x/GMCLIB/FLT/GMCLIB_Park_FLT/copyright2 ==

== system ammclib_bam_S32K14x/GMCLIB/FLT/GMCLIB_PwmIct_FLT/copyright ==

== system ammclib_bam_S32K14x/GMCLIB/FLT/GMCLIB_PwmIct_FLT/copyright2 ==

== system ammclib_bam_S32K14x/GMCLIB/FLT/GMCLIB_SvmSci_FLT/copyright ==

== system ammclib_bam_S32K14x/GMCLIB/FLT/GMCLIB_SvmSci_FLT/copyright2 ==

== system ammclib_bam_S32K14x/GMCLIB/FLT/GMCLIB_SvmStd_FLT/copyright ==

== system ammclib_bam_S32K14x/GMCLIB/FLT/GMCLIB_SvmStd_FLT/copyright2 ==

== system ammclib_bam_S32K14x/GMCLIB/FLT/GMCLIB_SvmU0n_FLT/copyright ==

== system ammclib_bam_S32K14x/GMCLIB/FLT/GMCLIB_SvmU0n_FLT/copyright2 ==

== system ammclib_bam_S32K14x/GMCLIB/FLT/GMCLIB_SvmU7n_FLT/copyright ==

== system ammclib_bam_S32K14x/GMCLIB/FLT/GMCLIB_SvmU7n_FLT/copyright2 ==

== system ammclib_bam_S32K14x/GMCLIB/FLT/GMCLIB_VRot_FLT/copyright ==

== system ammclib_bam_S32K14x/GMCLIB/FLT/GMCLIB_VRot_FLT/copyright2 ==

== system ammclib_bam_S32K14x/GMCLIB/FLT/GMCLIB_VUnit_FLT/copyright ==

== system ammclib_bam_S32K14x/GMCLIB/FLT/GMCLIB_VUnit_FLT/copyright2 ==

== system ammclib_bam_S32K14x/GMCLIB/FLT/GMCLIB_Vpol2xy_FLT/copyright ==

== system ammclib_bam_S32K14x/GMCLIB/FLT/GMCLIB_Vpol2xy_FLT/copyright2 ==

== system ammclib_bam_S32K14x/GMCLIB/FLT/GMCLIB_Vxy2pol_FLT/copyright ==

== system ammclib_bam_S32K14x/GMCLIB/FLT/GMCLIB_Vxy2pol_FLT/copyright2 ==

== system ammclib_bam_S32K14x/MLIB/F16/MLIB_AbsSat_F16/copyright ==

== system ammclib_bam_S32K14x/MLIB/F16/MLIB_AbsSat_F16/copyright2 ==

== system ammclib_bam_S32K14x/MLIB/F16/MLIB_Abs_F16/copyright ==

== system ammclib_bam_S32K14x/MLIB/F16/MLIB_Abs_F16/copyright2 ==

== system ammclib_bam_S32K14x/MLIB/F16/MLIB_AddSat_F16/copyright ==

== system ammclib_bam_S32K14x/MLIB/F16/MLIB_AddSat_F16/copyright2 ==

== system ammclib_bam_S32K14x/MLIB/F16/MLIB_Add_F16/copyright ==

== system ammclib_bam_S32K14x/MLIB/F16/MLIB_Add_F16/copyright2 ==

== system ammclib_bam_S32K14x/MLIB/F16/MLIB_ConvertPU_F16F32/copyright ==

== system ammclib_bam_S32K14x/MLIB/F16/MLIB_ConvertPU_F16F32/copyright2 ==

== system ammclib_bam_S32K14x/MLIB/F16/MLIB_ConvertPU_F16FLT/copyright ==

== system ammclib_bam_S32K14x/MLIB/F16/MLIB_ConvertPU_F16FLT/copyright2 ==

== system ammclib_bam_S32K14x/MLIB/F16/MLIB_Convert_F16F32/copyright ==

== system ammclib_bam_S32K14x/MLIB/F16/MLIB_Convert_F16F32/copyright2 ==

== system ammclib_bam_S32K14x/MLIB/F16/MLIB_Convert_F16FLT/copyright ==

== system ammclib_bam_S32K14x/MLIB/F16/MLIB_Convert_F16FLT/copyright2 ==

== system ammclib_bam_S32K14x/MLIB/F16/MLIB_DivSat_F16/copyright ==

== system ammclib_bam_S32K14x/MLIB/F16/MLIB_DivSat_F16/copyright2 ==

== system ammclib_bam_S32K14x/MLIB/F16/MLIB_Div_F16/copyright ==

== system ammclib_bam_S32K14x/MLIB/F16/MLIB_Div_F16/copyright2 ==

== system ammclib_bam_S32K14x/MLIB/F16/MLIB_MacSat_F16/copyright ==

== system ammclib_bam_S32K14x/MLIB/F16/MLIB_MacSat_F16/copyright2 ==

== system ammclib_bam_S32K14x/MLIB/F16/MLIB_Mac_F16/copyright ==

== system ammclib_bam_S32K14x/MLIB/F16/MLIB_Mac_F16/copyright2 ==

== system ammclib_bam_S32K14x/MLIB/F16/MLIB_Mnac_F16/copyright ==

== system ammclib_bam_S32K14x/MLIB/F16/MLIB_Mnac_F16/copyright2 ==

== system ammclib_bam_S32K14x/MLIB/F16/MLIB_Msu_F16/copyright ==

== system ammclib_bam_S32K14x/MLIB/F16/MLIB_Msu_F16/copyright2 ==

== system ammclib_bam_S32K14x/MLIB/F16/MLIB_MulSat_F16/copyright ==

== system ammclib_bam_S32K14x/MLIB/F16/MLIB_MulSat_F16/copyright2 ==

== system ammclib_bam_S32K14x/MLIB/F16/MLIB_Mul_F16/copyright ==

== system ammclib_bam_S32K14x/MLIB/F16/MLIB_Mul_F16/copyright2 ==

== system ammclib_bam_S32K14x/MLIB/F16/MLIB_NegSat_F16/copyright ==

== system ammclib_bam_S32K14x/MLIB/F16/MLIB_NegSat_F16/copyright2 ==

== system ammclib_bam_S32K14x/MLIB/F16/MLIB_Neg_F16/copyright ==

== system ammclib_bam_S32K14x/MLIB/F16/MLIB_Neg_F16/copyright2 ==

== system ammclib_bam_S32K14x/MLIB/F16/MLIB_Norm_F16/copyright ==

== system ammclib_bam_S32K14x/MLIB/F16/MLIB_Norm_F16/copyright2 ==

== system ammclib_bam_S32K14x/MLIB/F16/MLIB_RndSat_F16F32/copyright ==

== system ammclib_bam_S32K14x/MLIB/F16/MLIB_RndSat_F16F32/copyright2 ==

== system ammclib_bam_S32K14x/MLIB/F16/MLIB_Round_F16/copyright ==

== system ammclib_bam_S32K14x/MLIB/F16/MLIB_Round_F16/copyright2 ==

== system ammclib_bam_S32K14x/MLIB/F16/MLIB_ShBiSat_F16/copyright ==

== system ammclib_bam_S32K14x/MLIB/F16/MLIB_ShBiSat_F16/copyright2 ==

== system ammclib_bam_S32K14x/MLIB/F16/MLIB_ShBi_F16/copyright ==

== system ammclib_bam_S32K14x/MLIB/F16/MLIB_ShBi_F16/copyright2 ==

== system ammclib_bam_S32K14x/MLIB/F16/MLIB_ShLSat_F16/copyright ==

== system ammclib_bam_S32K14x/MLIB/F16/MLIB_ShLSat_F16/copyright2 ==

== system ammclib_bam_S32K14x/MLIB/F16/MLIB_ShL_F16/copyright ==

== system ammclib_bam_S32K14x/MLIB/F16/MLIB_ShL_F16/copyright2 ==

== system ammclib_bam_S32K14x/MLIB/F16/MLIB_ShR_F16/copyright ==

== system ammclib_bam_S32K14x/MLIB/F16/MLIB_ShR_F16/copyright2 ==

== system ammclib_bam_S32K14x/MLIB/F16/MLIB_SubSat_F16/copyright ==

== system ammclib_bam_S32K14x/MLIB/F16/MLIB_SubSat_F16/copyright2 ==

== system ammclib_bam_S32K14x/MLIB/F16/MLIB_Sub_F16/copyright ==

== system ammclib_bam_S32K14x/MLIB/F16/MLIB_Sub_F16/copyright2 ==

== system ammclib_bam_S32K14x/MLIB/F16/MLIB_VAdd_F16/copyright ==

== system ammclib_bam_S32K14x/MLIB/F16/MLIB_VAdd_F16/copyright2 ==

== system ammclib_bam_S32K14x/MLIB/F16/MLIB_VMac_F16/copyright ==

== system ammclib_bam_S32K14x/MLIB/F16/MLIB_VMac_F16/copyright2 ==

== system ammclib_bam_S32K14x/MLIB/F16/MLIB_VScale_F16/copyright ==

== system ammclib_bam_S32K14x/MLIB/F16/MLIB_VScale_F16/copyright2 ==

== system ammclib_bam_S32K14x/MLIB/F16/MLIB_VSub_F16/copyright ==

== system ammclib_bam_S32K14x/MLIB/F16/MLIB_VSub_F16/copyright2 ==

== system ammclib_bam_S32K14x/MLIB/F32/MLIB_AbsSat_F32/copyright ==

== system ammclib_bam_S32K14x/MLIB/F32/MLIB_AbsSat_F32/copyright2 ==

== system ammclib_bam_S32K14x/MLIB/F32/MLIB_Abs_F32/copyright ==

== system ammclib_bam_S32K14x/MLIB/F32/MLIB_Abs_F32/copyright2 ==

== system ammclib_bam_S32K14x/MLIB/F32/MLIB_AddSat_F32/copyright ==

== system ammclib_bam_S32K14x/MLIB/F32/MLIB_AddSat_F32/copyright2 ==

== system ammclib_bam_S32K14x/MLIB/F32/MLIB_Add_F32/copyright ==

== system ammclib_bam_S32K14x/MLIB/F32/MLIB_Add_F32/copyright2 ==

== system ammclib_bam_S32K14x/MLIB/F32/MLIB_ConvertPU_F32F16/copyright ==

== system ammclib_bam_S32K14x/MLIB/F32/MLIB_ConvertPU_F32F16/copyright2 ==

== system ammclib_bam_S32K14x/MLIB/F32/MLIB_ConvertPU_F32FLT/copyright ==

== system ammclib_bam_S32K14x/MLIB/F32/MLIB_ConvertPU_F32FLT/copyright2 ==

== system ammclib_bam_S32K14x/MLIB/F32/MLIB_Convert_F32F16/copyright ==

== system ammclib_bam_S32K14x/MLIB/F32/MLIB_Convert_F32F16/copyright2 ==

== system ammclib_bam_S32K14x/MLIB/F32/MLIB_Convert_F32FLT/copyright ==

== system ammclib_bam_S32K14x/MLIB/F32/MLIB_Convert_F32FLT/copyright2 ==

== system ammclib_bam_S32K14x/MLIB/F32/MLIB_DivSat_F32/copyright ==

== system ammclib_bam_S32K14x/MLIB/F32/MLIB_DivSat_F32/copyright2 ==

== system ammclib_bam_S32K14x/MLIB/F32/MLIB_Div_F32/copyright ==

== system ammclib_bam_S32K14x/MLIB/F32/MLIB_Div_F32/copyright2 ==

== system ammclib_bam_S32K14x/MLIB/F32/MLIB_MacSat_F32/copyright ==

== system ammclib_bam_S32K14x/MLIB/F32/MLIB_MacSat_F32/copyright2 ==

== system ammclib_bam_S32K14x/MLIB/F32/MLIB_Mac_F32/copyright ==

== system ammclib_bam_S32K14x/MLIB/F32/MLIB_Mac_F32/copyright2 ==

== system ammclib_bam_S32K14x/MLIB/F32/MLIB_Mnac_F32/copyright ==

== system ammclib_bam_S32K14x/MLIB/F32/MLIB_Mnac_F32/copyright2 ==

== system ammclib_bam_S32K14x/MLIB/F32/MLIB_Msu_F32/copyright ==

== system ammclib_bam_S32K14x/MLIB/F32/MLIB_Msu_F32/copyright2 ==

== system ammclib_bam_S32K14x/MLIB/F32/MLIB_MulSat_F32/copyright ==

== system ammclib_bam_S32K14x/MLIB/F32/MLIB_MulSat_F32/copyright2 ==

== system ammclib_bam_S32K14x/MLIB/F32/MLIB_Mul_F32/copyright ==

== system ammclib_bam_S32K14x/MLIB/F32/MLIB_Mul_F32/copyright2 ==

== system ammclib_bam_S32K14x/MLIB/F32/MLIB_NegSat_F32/copyright ==

== system ammclib_bam_S32K14x/MLIB/F32/MLIB_NegSat_F32/copyright2 ==

== system ammclib_bam_S32K14x/MLIB/F32/MLIB_Neg_F32/copyright ==

== system ammclib_bam_S32K14x/MLIB/F32/MLIB_Neg_F32/copyright2 ==

== system ammclib_bam_S32K14x/MLIB/F32/MLIB_Norm_F32/copyright ==

== system ammclib_bam_S32K14x/MLIB/F32/MLIB_Norm_F32/copyright2 ==

== system ammclib_bam_S32K14x/MLIB/F32/MLIB_Round_F32/copyright ==

== system ammclib_bam_S32K14x/MLIB/F32/MLIB_Round_F32/copyright2 ==

== system ammclib_bam_S32K14x/MLIB/F32/MLIB_ShBiSat_F32/copyright ==

== system ammclib_bam_S32K14x/MLIB/F32/MLIB_ShBiSat_F32/copyright2 ==

== system ammclib_bam_S32K14x/MLIB/F32/MLIB_ShBi_F32/copyright ==

== system ammclib_bam_S32K14x/MLIB/F32/MLIB_ShBi_F32/copyright2 ==

== system ammclib_bam_S32K14x/MLIB/F32/MLIB_ShLSat_F32/copyright ==

== system ammclib_bam_S32K14x/MLIB/F32/MLIB_ShLSat_F32/copyright2 ==

== system ammclib_bam_S32K14x/MLIB/F32/MLIB_ShL_F32/copyright ==

== system ammclib_bam_S32K14x/MLIB/F32/MLIB_ShL_F32/copyright2 ==

== system ammclib_bam_S32K14x/MLIB/F32/MLIB_ShR_F32/copyright ==

== system ammclib_bam_S32K14x/MLIB/F32/MLIB_ShR_F32/copyright2 ==

== system ammclib_bam_S32K14x/MLIB/F32/MLIB_SubSat_F32/copyright ==

== system ammclib_bam_S32K14x/MLIB/F32/MLIB_SubSat_F32/copyright2 ==

== system ammclib_bam_S32K14x/MLIB/F32/MLIB_Sub_F32/copyright ==

== system ammclib_bam_S32K14x/MLIB/F32/MLIB_Sub_F32/copyright2 ==

== system ammclib_bam_S32K14x/MLIB/F32/MLIB_VAdd_F32/copyright ==

== system ammclib_bam_S32K14x/MLIB/F32/MLIB_VAdd_F32/copyright2 ==

== system ammclib_bam_S32K14x/MLIB/F32/MLIB_VMac_F32/copyright ==

== system ammclib_bam_S32K14x/MLIB/F32/MLIB_VMac_F32/copyright2 ==

== system ammclib_bam_S32K14x/MLIB/F32/MLIB_VScale_F32/copyright ==

== system ammclib_bam_S32K14x/MLIB/F32/MLIB_VScale_F32/copyright2 ==

== system ammclib_bam_S32K14x/MLIB/F32/MLIB_VSub_F32/copyright ==

== system ammclib_bam_S32K14x/MLIB/F32/MLIB_VSub_F32/copyright2 ==

== system ammclib_bam_S32K14x/MLIB/F32F16F16/MLIB_MacSat_F32F16F16/copyright ==

== system ammclib_bam_S32K14x/MLIB/F32F16F16/MLIB_MacSat_F32F16F16/copyright2 ==

== system ammclib_bam_S32K14x/MLIB/F32F16F16/MLIB_Mac_F32F16F16/copyright ==

== system ammclib_bam_S32K14x/MLIB/F32F16F16/MLIB_Mac_F32F16F16/copyright2 ==

== system ammclib_bam_S32K14x/MLIB/F32F16F16/MLIB_Mnac_F32F16F16/copyright ==

== system ammclib_bam_S32K14x/MLIB/F32F16F16/MLIB_Mnac_F32F16F16/copyright2 ==

== system ammclib_bam_S32K14x/MLIB/F32F16F16/MLIB_Msu_F32F16F16/copyright ==

== system ammclib_bam_S32K14x/MLIB/F32F16F16/MLIB_Msu_F32F16F16/copyright2 ==

== system ammclib_bam_S32K14x/MLIB/F32F16F16/MLIB_MulSat_F32F16F16/copyright ==

== system ammclib_bam_S32K14x/MLIB/F32F16F16/MLIB_MulSat_F32F16F16/copyright2 ==

== system ammclib_bam_S32K14x/MLIB/F32F16F16/MLIB_Mul_F32F16F16/copyright ==

== system ammclib_bam_S32K14x/MLIB/F32F16F16/MLIB_Mul_F32F16F16/copyright2 ==

== system ammclib_bam_S32K14x/MLIB/F32F16F16/MLIB_VMac_F32F16F16/copyright ==

== system ammclib_bam_S32K14x/MLIB/F32F16F16/MLIB_VMac_F32F16F16/copyright2 ==

== system ammclib_bam_S32K14x/MLIB/FLT/MLIB_Abs_FLT/copyright ==

== system ammclib_bam_S32K14x/MLIB/FLT/MLIB_Abs_FLT/copyright2 ==

== system ammclib_bam_S32K14x/MLIB/FLT/MLIB_Add_FLT/copyright ==

== system ammclib_bam_S32K14x/MLIB/FLT/MLIB_Add_FLT/copyright2 ==

== system ammclib_bam_S32K14x/MLIB/FLT/MLIB_ConvertPU_FLTF16/copyright ==

== system ammclib_bam_S32K14x/MLIB/FLT/MLIB_ConvertPU_FLTF16/copyright2 ==

== system ammclib_bam_S32K14x/MLIB/FLT/MLIB_ConvertPU_FLTF32/copyright ==

== system ammclib_bam_S32K14x/MLIB/FLT/MLIB_ConvertPU_FLTF32/copyright2 ==

== system ammclib_bam_S32K14x/MLIB/FLT/MLIB_Convert_FLTF16/copyright ==

== system ammclib_bam_S32K14x/MLIB/FLT/MLIB_Convert_FLTF16/copyright2 ==

== system ammclib_bam_S32K14x/MLIB/FLT/MLIB_Convert_FLTF32/copyright ==

== system ammclib_bam_S32K14x/MLIB/FLT/MLIB_Convert_FLTF32/copyright2 ==

== system ammclib_bam_S32K14x/MLIB/FLT/MLIB_Div_FLT/copyright ==

== system ammclib_bam_S32K14x/MLIB/FLT/MLIB_Div_FLT/copyright2 ==

== system ammclib_bam_S32K14x/MLIB/FLT/MLIB_Mac_FLT/copyright ==

== system ammclib_bam_S32K14x/MLIB/FLT/MLIB_Mac_FLT/copyright2 ==

== system ammclib_bam_S32K14x/MLIB/FLT/MLIB_Mnac_FLT/copyright ==

== system ammclib_bam_S32K14x/MLIB/FLT/MLIB_Mnac_FLT/copyright2 ==

== system ammclib_bam_S32K14x/MLIB/FLT/MLIB_Msu_FLT/copyright ==

== system ammclib_bam_S32K14x/MLIB/FLT/MLIB_Msu_FLT/copyright2 ==

== system ammclib_bam_S32K14x/MLIB/FLT/MLIB_Mul_FLT/copyright ==

== system ammclib_bam_S32K14x/MLIB/FLT/MLIB_Mul_FLT/copyright2 ==

== system ammclib_bam_S32K14x/MLIB/FLT/MLIB_Neg_FLT/copyright ==

== system ammclib_bam_S32K14x/MLIB/FLT/MLIB_Neg_FLT/copyright2 ==

== system ammclib_bam_S32K14x/MLIB/FLT/MLIB_Sub_FLT/copyright ==

== system ammclib_bam_S32K14x/MLIB/FLT/MLIB_Sub_FLT/copyright2 ==

== system ammclib_bam_S32K14x/MLIB/FLT/MLIB_VAdd_FLT/copyright ==

== system ammclib_bam_S32K14x/MLIB/FLT/MLIB_VAdd_FLT/copyright2 ==

== system ammclib_bam_S32K14x/MLIB/FLT/MLIB_VMac_FLT/copyright ==

== system ammclib_bam_S32K14x/MLIB/FLT/MLIB_VMac_FLT/copyright2 ==

== system ammclib_bam_S32K14x/MLIB/FLT/MLIB_VScale_FLT/copyright ==

== system ammclib_bam_S32K14x/MLIB/FLT/MLIB_VScale_FLT/copyright2 ==

== system ammclib_bam_S32K14x/MLIB/FLT/MLIB_VSub_FLT/copyright ==

== system ammclib_bam_S32K14x/MLIB/FLT/MLIB_VSub_FLT/copyright2 ==
